simulink subsystem "MacPhersonFrntSolidAxleMidlRearSusp"  (R2023b)
settings: Solver=VariableStepAuto  StartTime=0.0  StopTime=10.0  RelTol=1e-3
undefined symbols (not defined in the file): PlntVehCGHgtAxl
libraries: sharedtransform x4, vehdynlibsuspension x2, autolibutils x2, matrix_library x1
settings Model: ModifiedByFormat=The MathWorks, Inc.  Creator=The MathWorks, Inc.  LastModifiedBy=The MathWorks, Inc.
settings OptimizationCC: ReuseModelBlockBuffer=off

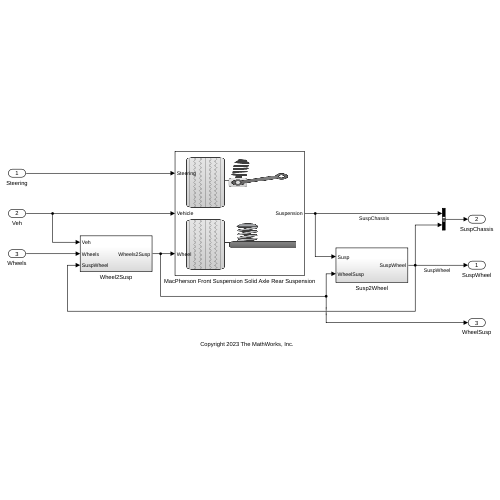
[thumbnail: Simulink's stored preview of the top-level diagram]
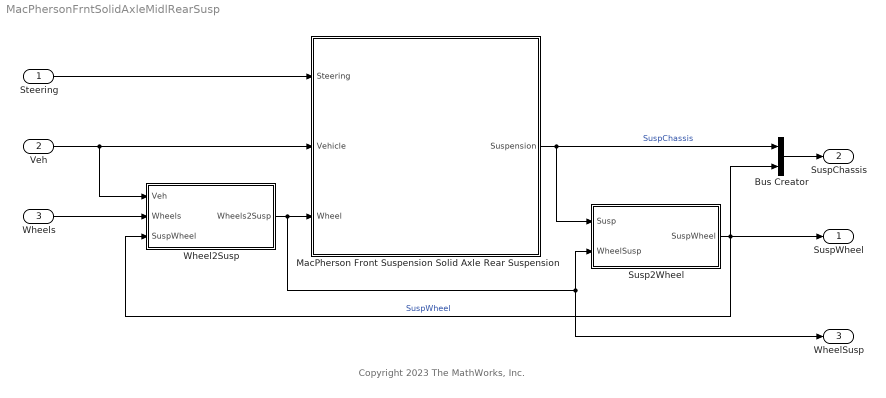
== system MacPhersonFrntSolidAxleMidlRearSusp ==
  note: Copyright 2023 The MathWorks, Inc.
  Steering : Inport
  Veh : Inport  Port=2
  Wheels : Inport  Port=3
  Bus Creator : BusCreator  Inputs=2
  MacPherson Front Suspension Solid Axle Rear Suspension : Subsystem  VariantControl=MacPherson Front Suspension Solid Axle Rear Suspension
      mask Display: image([imread('suspmacp.png');imread('suspsacoil.png')]);
  Susp2Wheel : Subsystem
  Wheel2Susp : Subsystem
  SuspWheel : Outport
  SuspChassis : Outport  Port=2
  WheelSusp : Outport  Port=3
  wires:
  Bus Creator/1 -> SuspChassis/1
  Wheel2Susp/1(Wheels2Susp) -> Susp2Wheel/2(WheelSusp), WheelSusp/1, MacPherson Front Suspension Solid Axle Rear Suspension/3(Wheel)
  Susp2Wheel/1(SuspWheel) -> SuspWheel/1, Bus Creator/2, Wheel2Susp/3(SuspWheel)  "SuspWheel"
  Wheels/1 -> Wheel2Susp/2(Wheels)
  Steering/1 -> MacPherson Front Suspension Solid Axle Rear Suspension/1(Steering)
  Veh/1 -> Wheel2Susp/1(Veh), MacPherson Front Suspension Solid Axle Rear Suspension/2(Vehicle)
  MacPherson Front Suspension Solid Axle Rear Suspension/1(Suspension) -> Susp2Wheel/1(Susp), Bus Creator/1  "SuspChassis"

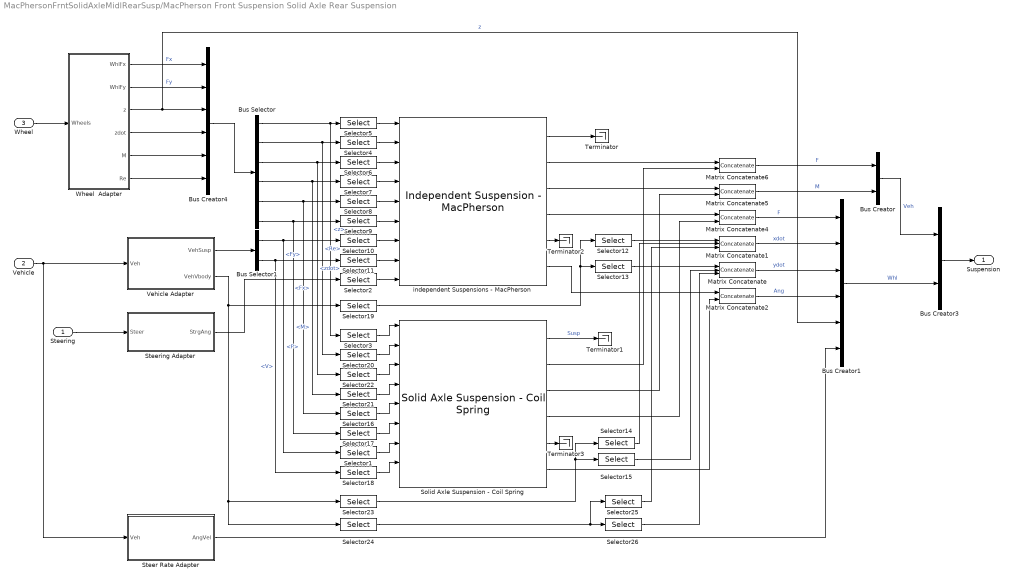
== system MacPhersonFrntSolidAxleMidlRearSusp/MacPherson Front Suspension Solid Axle Rear Suspension ==
  Steering : Inport
  Vehicle : Inport  Port=2
  Wheel : Inport  Port=3
  Bus Creator : BusCreator  Inputs=2
  Bus Creator1 : BusCreator  Inputs=6
  Bus Creator3 : BusCreator  Inputs=2
  Bus Creator4 : BusCreator  Inputs=6
  Bus Selector : BusSelector  OutputSignals=z,Re,zdot,Fx,Fy,M
  Bus Selector1 : BusSelector  OutputSignals=P,V
  Matrix Concatenate : Concatenate  NumInputs=3  Mode=Multidimensional array  ConcatenateDimension=2
  Matrix Concatenate1 : Concatenate  NumInputs=3  Mode=Multidimensional array  ConcatenateDimension=2
  Matrix Concatenate{2,4..6} (4 alike) : Concatenate  Mode=Multidimensional array  ConcatenateDimension=2
  Selector1 : Selector  NumberOfDimensions=2  IndexOptions=Select all,Index vector (dialog)  Indices=[1 2],[3 4 5 6]  OutputSizes=1,1
  Selector{9..11,19} (4 alike) : Selector  NumberOfDimensions=2  IndexOptions=Select all,Index vector (dialog)  Indices=[1 2],[1 2]  OutputSizes=1,1
  Selector12 : Selector  NumberOfDimensions=2  InputPortWidth=3  IndexOptions=Index vector (dialog),Select all  Indices=1,1  OutputSizes=1,1
  Selector13 : Selector  NumberOfDimensions=2  InputPortWidth=3  IndexOptions=Index vector (dialog),Select all  Indices=2,1  OutputSizes=1,1
  Selector14 : Selector  NumberOfDimensions=2  InputPortWidth=3  IndexOptions=Index vector (dialog),Select all  Indices=1,1  OutputSizes=1,1
  Selector15 : Selector  NumberOfDimensions=2  InputPortWidth=3  IndexOptions=Index vector (dialog),Select all  Indices=2,1  OutputSizes=1,1
  Selector{3,16,20..22} (5 alike) : Selector  IndexOptions=Index vector (dialog)  Indices=[3 4 5 6]  OutputSizes=1
  Selector17 : Selector  NumberOfDimensions=2  IndexOptions=Select all,Index vector (dialog)  Indices=[1 2],[3 4 5 6]  OutputSizes=1,1
  Selector18 : Selector  NumberOfDimensions=2  IndexOptions=Select all,Index vector (dialog)  Indices=[1 2],[3 4 5 6]  OutputSizes=1,1
  Selector2 : Selector  IndexOptions=Index vector (dialog)  Indices=[1 2]  OutputSizes=1
  Selector23 : Selector  NumberOfDimensions=2  IndexOptions=Select all,Index vector (dialog)  Indices=[1 2],[3 4]  OutputSizes=1,1
  Selector24 : Selector  NumberOfDimensions=2  IndexOptions=Select all,Index vector (dialog)  Indices=[1 2],[5 6]  OutputSizes=1,1
  Selector25 : Selector  NumberOfDimensions=2  InputPortWidth=3  IndexOptions=Index vector (dialog),Select all  Indices=1,1  OutputSizes=1,1
  Selector26 : Selector  NumberOfDimensions=2  InputPortWidth=3  IndexOptions=Index vector (dialog),Select all  Indices=2,1  OutputSizes=1,1
  Selector{4..8} (5 alike) : Selector  InputPortWidth=6  IndexOptions=Index vector (dialog)  Indices=[1 2]  OutputSizes=1
  Solid Axle Suspension - Coil Spring : vehdynlibsuspension/Solid Axle Suspension - Coil Spring  NumAxl=2  NumWhlsByAxl=[2 2]  StrgEnByAxl=[0 0]  WhlNumVec="[1  2  1  2]"  AxleNumVec="[1  1  2  2]"  SuspTypesByAxle="[1  1]"  SuspImage=suspsacoil.png  AxlIxx=PlntSpSARollInertia  AxlM=PlntSpSAAxleMass  TrackCoords="[zeros(1,4);1.575*[1 -1  1 -1]/2;zeros(1,4)]"  SuspCoords="[zeros(1,4);1.575*[1 -1  1 -1]/2;zeros(1,4)]"  KzWhlAxl=PlntSpSAAxleWheelStiffness  F0zWhlAxl=PlntSpSAAxleWheelPreload  CzWhlAxl=PlntSpSAAxleWheelDamping  IdealSuspEn=on  IdealSuspAxles="[1  2]"  Kz=PlntSpSAStiffness  F0z=PlntSpSAPreload  Cz=PlntSpSADamping  Hmax=PlntSpSAMaxHeight  Toe=PlntSpSAStatToe  RollStrgSlp=0.  ToeStrgSlp=0  Caster=PlntSpSAStatCaster  CasterHslp=0.  CasterStrgSlp=0.01  Camber=PlntSpSAStatCamber  CamberHslp=0.  CamberStrgSlp=0.01  StrgHgtSlp=0.1432  MappedSuspEn=off  MappedSuspAxles="[1  2]"  f_susp_axl_bp=[1 2]  f_susp_dz_bp=[-0.15 -0.14 -0.13 -0.12 -0.11 -0.10 -0.09 -0.08 -0.07 -0.06 -0.05 -0.04 -0.03 -0.02 -0.01 0.00 0.01 0.02 0.03 0.04 0.05 0.06 0.07 0.08 0.09 0.10 0.11 0.12 0.13 0.14 0.15]  f_susp_dzdot_bp=[-0.15 -0.14 -0.13 -0.12 -0.11 -0.10 -0.09 -0.08 -0.07 -0.06 -0.05 -0.04 -0.03 -0.02 -0.01 0.00 0.01 0.02 0.03 0.04 0.05 0.06 0.07 0.08 0.09 0.10 0.11 0.12 0.13 0.14 0.15]  f_susp_fmz=zeros(31,31,61,2,4)  f_susp_geom=zeros(31,61,2,3)  f_susp_strgdelta_bp=[-30,-29,-28,-27,-26,-25,-24,-23,-22,-21,-20,-19,-18,-17,-16,-15,-14,-13,-12,-11,-10,-9,-8,-7,-6,-5,-4,-3,-2,-1,0,1,2,3,4,5,6,7,8,9,10,11,12,13,14,15,16,17,18,19,20,21,22,23,24,25,26,27,28,29,30]
  Steer Rate Adapter : Subsystem
  Steering Adapter : Subsystem
  Terminator{,1..3} (4 alike) : Terminator
  Vehicle Adapter : Subsystem
  Wheel  Adapter : Subsystem
  independent Suspensions - MacPherson : vehdynlibsuspension/Independent Suspension - MacPherson  ActiveDampEn=off  NumAxl=1  NumWhlsByAxl=2  StrgEnByAxl=1  AntiSwayEnByAxl=1  WhlNumVec="[1  2]"  AxleNumVec="[1  1]"  SuspTypesByAxle=[1]  SuspImage=suspmacp.png  IdealSuspEn=on  IdealSuspAxles=[1]  Kz=PlntSpMSStiffness  F0z=PlntSpMSPreload  Cz=PlntSpMSDamping  Hmax=PlntSpMSMaxHeight  f_act_susp_cz=[10000 10000;10000 10000]  f_act_susp_duty_bpt=[0 1]  f_act_susp_zdot_bpt=[-1 1]  Toe=PlntSpMSStatToe  RollStrgSlp=0.  ToeStrgSlp=0.  Caster=PlntSpMSStatCaster  CasterHslp=0.  CasterStrgSlp=0.  Camber=PlntSpMSStatCamber  CamberHslp=0.  CamberStrgSlp=0.  StrgHgtSlp=PlntSpMSHeightVsSteer  MappedSuspEn=off  MappedSuspAxles="[1  2]"  f_susp_axl_bp=[1 2]  f_susp_dz_bp=[-0.15 -0.14 -0.13 -0.12 -0.11 -0.10 -0.09 -0.08 -0.07 -0.06 -0.05 -0.04 -0.03 -0.02 -0.01 0.00 0.01 0.02 0.03 0.04 0.05 0.06 0.07 0.08 0.09 0.10 0.11 0.12 0.13 0.14 0.15]  f_susp_dzdot_bp=[-0.15 -0.14 -0.13 -0.12 -0.11 -0.10 -0.09 -0.08 -0.07 -0.06 -0.05 -0.04 -0.03 -0.02 -0.01 0.00 0.01 0.02 0.03 0.04 0.05 0.06 0.07 0.08 0.09 0.10 0.11 0.12 0.13 0.14 0.15]  f_susp_fmz=zeros(31,31,61,2,4)  f_susp_geom=zeros(31,61,2,3)  f_susp_strgdelta_bp=[-30,-29,-28,-27,-26,-25,-24,-23,-22,-21,-20,-19,-18,-17,-16,-15,-14,-13,-12,-11,-10,-9,-8,-7,-6,-5,-4,-3,-2,-1,0,1,2,3,4,5,6,7,8,9,10,11,12,13,14,15,16,17,18,19,20,21,22,23,24,25,26,27,28,29,30]  AntiSwayR=PlntSpMSAntiSwayRadius  AntiSwayNtrlAng=PlntSpMSAntiSwayNeutralAngle  AntiSwayTrsK=PlntSpMSAntiSwayTorsionStiffness
  Suspension : Outport  VectorParamsAs1DForOutWhenUnconnected=off
  wires:
  Selector26/1 -> Matrix Concatenate/3
  Selector25/1 -> Matrix Concatenate1/3
  Selector24/1 -> Selector25/1, Selector26/1
  Selector23/1 -> Selector14/1, Selector15/1
  Selector19/1 -> Selector13/1, Selector12/1
  Solid Axle Suspension - Coil Spring/5 -> Terminator3/1
  independent Suspensions - MacPherson/5 -> Terminator2/1
  Steer Rate Adapter/1(AngVel) -> Bus Creator1/6
  Vehicle Adapter/2(VehVbody) -> Selector19/1, Selector23/1, Selector24/1
  Solid Axle Suspension - Coil Spring/1 -> Terminator1/1  "Susp"
  Bus Selector/3 -> Selector6/1, Selector22/1  "<zdot>"
  Selector22/1 -> Solid Axle Suspension - Coil Spring/3
  Vehicle/1 -> Steer Rate Adapter/1(Veh), Vehicle Adapter/1(Veh)
  Solid Axle Suspension - Coil Spring/3 -> Matrix Concatenate5/2
  Selector21/1 -> Solid Axle Suspension - Coil Spring/4
  Wheel  Adapter/6(Re) -> Bus Creator4/6
  Selector20/1 -> Solid Axle Suspension - Coil Spring/2
  Selector18/1 -> Solid Axle Suspension - Coil Spring/8
  Selector1/1 -> Solid Axle Suspension - Coil Spring/7
  Selector17/1 -> Solid Axle Suspension - Coil Spring/6
  Selector16/1 -> Solid Axle Suspension - Coil Spring/5
  Solid Axle Suspension - Coil Spring/2 -> Matrix Concatenate6/2
  Matrix Concatenate6/1 -> Bus Creator/1  "F"
  Matrix Concatenate5/1 -> Bus Creator/2  "M"
  Solid Axle Suspension - Coil Spring/4 -> Matrix Concatenate4/2
  Matrix Concatenate4/1 -> Bus Creator1/1  "F"
  Solid Axle Suspension - Coil Spring/6 -> Matrix Concatenate2/2
  Matrix Concatenate2/1 -> Bus Creator1/4  "Ang"
  Selector14/1 -> Matrix Concatenate1/2
  Matrix Concatenate1/1 -> Bus Creator1/2  "xdot"
  Selector15/1 -> Matrix Concatenate/2
  Selector13/1 -> Matrix Concatenate/1
  Selector11/1 -> independent Suspensions - MacPherson/8
  Selector10/1 -> independent Suspensions - MacPherson/7
  Selector9/1 -> independent Suspensions - MacPherson/6
  Selector8/1 -> independent Suspensions - MacPherson/5
  Selector7/1 -> independent Suspensions - MacPherson/4
  Selector6/1 -> independent Suspensions - MacPherson/3
  Selector5/1 -> independent Suspensions - MacPherson/1
  Selector4/1 -> independent Suspensions - MacPherson/2
  Selector3/1 -> Solid Axle Suspension - Coil Spring/1
  Selector2/1 -> independent Suspensions - MacPherson/9
  Bus Selector/2 -> Selector4/1, Selector20/1  "<Re>"
  Wheel  Adapter/5(M) -> Bus Creator4/5
  Wheel  Adapter/4(zdot) -> Bus Creator4/4
  Wheel  Adapter/3(z) -> Bus Creator4/3, Bus Creator1/5  "z"
  Wheel/1 -> Wheel  Adapter/1(Wheels)
  Wheel  Adapter/1(WhlFx) -> Bus Creator4/1  "Fx"
  Wheel  Adapter/2(WhlFy) -> Bus Creator4/2  "Fy"
  Bus Creator4/1 -> Bus Selector/1
  Steering Adapter/1(StrgAng) -> Selector2/1
  Bus Creator/1 -> Bus Creator3/1  "Veh"
  independent Suspensions - MacPherson/3 -> Matrix Concatenate5/1
  independent Suspensions - MacPherson/2 -> Matrix Concatenate6/1
  Vehicle Adapter/1(VehSusp) -> Bus Selector1/1
  Bus Selector/4 -> Selector21/1, Selector7/1  "<Fx>"
  independent Suspensions - MacPherson/1 -> Terminator/1
  independent Suspensions - MacPherson/4 -> Matrix Concatenate4/1
  Selector12/1 -> Matrix Concatenate1/1
  independent Suspensions - MacPherson/6 -> Matrix Concatenate2/1
  Matrix Concatenate/1 -> Bus Creator1/3  "ydot"
  Bus Selector1/1 -> Selector1/1, Selector10/1  "<P>"
  Steering/1 -> Steering Adapter/1(Steer)
  Bus Selector/1 -> Selector5/1, Selector3/1  "<z>"
  Bus Selector/5 -> Selector16/1, Selector8/1  "<Fy>"
  Bus Selector/6 -> Selector17/1, Selector9/1  "<M>"
  Bus Selector1/2 -> Selector18/1, Selector11/1  "<V>"
  Bus Creator1/1 -> Bus Creator3/2  "Whl"
  Bus Creator3/1 -> Suspension/1

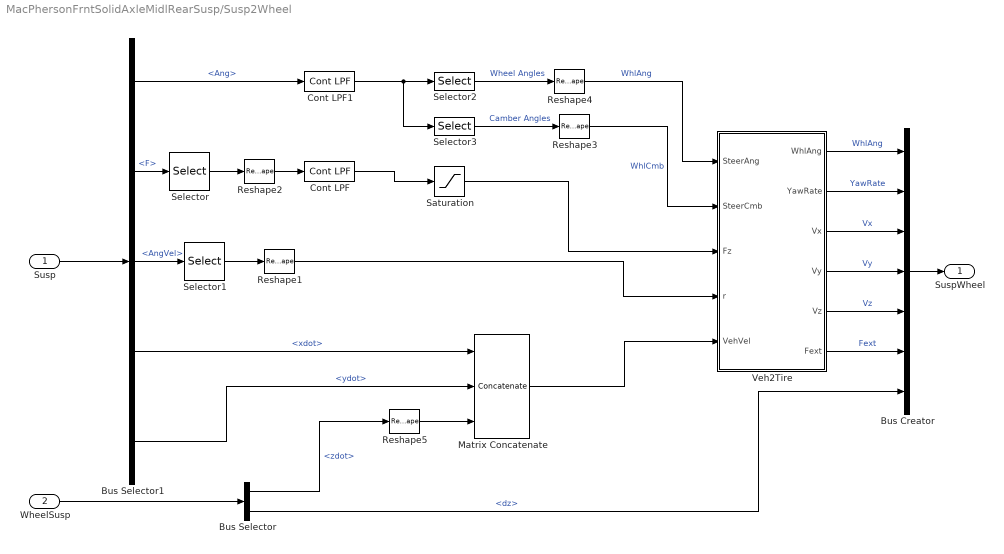
== system MacPhersonFrntSolidAxleMidlRearSusp/Susp2Wheel ==
  Susp : Inport
  WheelSusp : Inport  Port=2
  Bus Creator : BusCreator  Inputs=7
  Bus Selector : BusSelector  OutputSignals=SuspFrame.zdot,SuspFrame.dz
  Bus Selector1 : BusSelector  OutputSignals=Whl.Ang,Whl.F,Whl.AngVel,Whl.xdot,Whl.ydot
  Cont LPF : autolibutils/Cont LPF  wc=100*2*pi  AbsoluteTolerance=auto  aMode=2
  Cont LPF1 : autolibutils/Cont LPF  wc=100*2*pi  AbsoluteTolerance=auto  aMode=2
  Matrix Concatenate : Concatenate  NumInputs=3  Mode=Multidimensional array
  Reshape{1..4} (4 alike) : Reshape
  Reshape5 : Reshape  OutputDimensionality=Row vector (2-D)
  Saturation : Saturate  UpperLimit=inf  LowerLimit=-10*9.81*2000  ZeroCross=off
  Selector : Selector  NumberOfDimensions=2  InputPortWidth=3  IndexOptions=Index vector (dialog),Select all  Indices=[3],1  OutputSizes=1,1
  Selector1 : Selector  NumberOfDimensions=2  InputPortWidth=1  IndexOptions=Index vector (dialog),Select all  Indices=[3],1  OutputSizes=1,1
  Selector2 : Selector  NumberOfDimensions=2  InputPortWidth=3  IndexOptions=Index vector (dialog),Select all  Indices=3,1  OutputSizes=1,1
  Selector3 : Selector  NumberOfDimensions=2  InputPortWidth=3  IndexOptions=Index vector (dialog),Select all  Indices=1,1  OutputSizes=1,1
  Veh2Tire : Subsystem
  SuspWheel : Outport
  wires:
  Bus Creator/1 -> SuspWheel/1
  Bus Selector/1 -> Reshape5/1  "<zdot>"
  Veh2Tire/3(Vx) -> Bus Creator/3  "Vx"
  Veh2Tire/4(Vy) -> Bus Creator/4  "Vy"
  Susp/1 -> Bus Selector1/1
  Veh2Tire/5(Vz) -> Bus Creator/5  "Vz"
  Bus Selector1/1 -> Cont LPF1/1  "<Ang>"
  Reshape5/1 -> Matrix Concatenate/3
  WheelSusp/1 -> Bus Selector/1
  Cont LPF/1 -> Saturation/1
  Selector/1 -> Reshape2/1
  Matrix Concatenate/1 -> Veh2Tire/5(VehVel)
  Saturation/1 -> Veh2Tire/3(Fz)
  Selector1/1 -> Reshape1/1
  Veh2Tire/6(Fext) -> Bus Creator/6  "Fext"
  Bus Selector1/5 -> Matrix Concatenate/2  "<ydot>"
  Bus Selector1/3 -> Selector1/1  "<AngVel>"
  Bus Selector1/4 -> Matrix Concatenate/1  "<xdot>"
  Reshape4/1 -> Veh2Tire/1(SteerAng)  "WhlAng"
  Veh2Tire/1(WhlAng) -> Bus Creator/1  "WhlAng"
  Reshape3/1 -> Veh2Tire/2(SteerCmb)  "WhlCmb"
  Selector3/1 -> Reshape3/1  "Camber Angles"
  Reshape2/1 -> Cont LPF/1
  Selector2/1 -> Reshape4/1  "Wheel Angles"
  Reshape1/1 -> Veh2Tire/4(r)
  Cont LPF1/1 -> Selector3/1, Selector2/1
  Bus Selector1/2 -> Selector/1  "<F>"
  Veh2Tire/2(YawRate) -> Bus Creator/2  "YawRate"
  Bus Selector/2 -> Bus Creator/7  "<dz>"

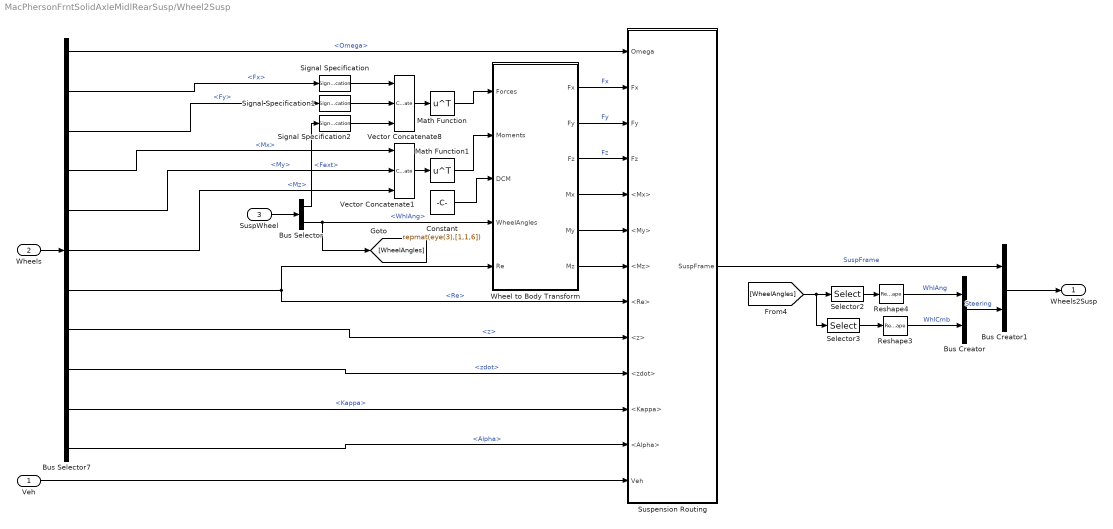
== system MacPhersonFrntSolidAxleMidlRearSusp/Wheel2Susp ==
  Veh : Inport
  Wheels : Inport  Port=2
  SuspWheel : Inport  Port=3
  Bus Creator : BusCreator  Inputs=2
  Bus Creator1 : BusCreator  Inputs=2
  Bus Selector : BusSelector  OutputSignals=Fext,WhlAng
  Bus Selector7 : BusSelector  OutputSignals=Wheels.Omega,Wheels.Fx,Wheels.Fy,Wheels.Mx,Wheels.My,Wheels.Mz,Wheels.Re,Wheels.z,Wheels.zdot,Wheels.Kappa,Wheels.Alpha
  Constant : Constant  Value=repmat(eye(3),[1,1,6])
  Math Function : Math  Operator=transpose  SignedPower=on
  Math Function1 : Math  Operator=transpose  SignedPower=on
  Reshape3 : Reshape
  Reshape4 : Reshape
  Selector2 : Selector  NumberOfDimensions=2  InputPortWidth=3  IndexOptions=Index vector (dialog),Select all  Indices=3,1  OutputSizes=1,1
  Selector3 : Selector  NumberOfDimensions=2  InputPortWidth=3  IndexOptions=Index vector (dialog),Select all  Indices=1,1  OutputSizes=1,1
  Signal Specification : SignalSpecification  Dimensions=6
  Signal Specification1 : SignalSpecification  Dimensions=6
  Signal Specification2 : SignalSpecification  Dimensions=6
  Suspension Routing : Subsystem
  Vector Concatenate1 : Concatenate  NumInputs=3  Mode=Multidimensional array  ConcatenateDimension=2
  Vector Concatenate8 : Concatenate  NumInputs=3  Mode=Multidimensional array  ConcatenateDimension=2
  Wheel to Body Transform : Subsystem
  Wheels2Susp : Outport  VectorParamsAs1DForOutWhenUnconnected=off
  wires:
  Bus Selector7/11 -> Suspension Routing/12(<Alpha>)  "<Alpha>"
  Bus Selector7/10 -> Suspension Routing/11(<Kappa>)  "<Kappa>"
  Bus Selector7/9 -> Suspension Routing/10(<zdot>)  "<zdot>"
  Bus Selector7/8 -> Suspension Routing/9(<z>)  "<z>"
  Bus Selector7/7 -> Suspension Routing/8(<Re>), Wheel to Body Transform/5(Re)  "<Re>"
  Bus Selector7/6 -> Vector Concatenate1/3  "<Mz>"
  Bus Selector7/5 -> Vector Concatenate1/2  "<My>"
  Bus Selector7/4 -> Vector Concatenate1/1  "<Mx>"
  Bus Selector7/3 -> Signal Specification1/1  "<Fy>"
  Bus Selector7/2 -> Signal Specification/1  "<Fx>"
  Bus Selector7/1 -> Suspension Routing/1(Omega)  "<Omega>"
  Constant/1 -> Wheel to Body Transform/3(DCM)
  Math Function1/1 -> Wheel to Body Transform/2(Moments)
  Vector Concatenate1/1 -> Math Function1/1
  Wheel to Body Transform/6(Mz) -> Suspension Routing/7(<Mz>)
  Wheel to Body Transform/5(My) -> Suspension Routing/6(<My>)
  Wheel to Body Transform/4(Mx) -> Suspension Routing/5(<Mx>)
  Selector3/1 -> Reshape3/1
  [WheelAngles] -> Selector3/1, Selector2/1
  Selector2/1 -> Reshape4/1
  Signal Specification2/1 -> Vector Concatenate8/3
  Bus Selector/1 -> Signal Specification2/1  "<Fext>"
  SuspWheel/1 -> Bus Selector/1
  Wheel to Body Transform/2(Fy) -> Suspension Routing/3(Fy)  "Fy"
  Wheel to Body Transform/1(Fx) -> Suspension Routing/2(Fx)  "Fx"
  Vector Concatenate8/1 -> Math Function/1
  Math Function/1 -> Wheel to Body Transform/1(Forces)
  Wheels/1 -> Bus Selector7/1
  Bus Selector/2 -> Wheel to Body Transform/4(WheelAngles), [WheelAngles]  "<WhlAng>"
  Wheel to Body Transform/3(Fz) -> Suspension Routing/4(Fz)  "Fz"
  Reshape4/1 -> Bus Creator/1  "WhlAng"
  Bus Creator1/1 -> Wheels2Susp/1
  Suspension Routing/1(SuspFrame) -> Bus Creator1/1  "SuspFrame"
  Reshape3/1 -> Bus Creator/2  "WhlCmb"
  Bus Creator/1 -> Bus Creator1/2  "Steering"
  Veh/1 -> Suspension Routing/13(Veh)
  Signal Specification/1 -> Vector Concatenate8/1
  Signal Specification1/1 -> Vector Concatenate8/2

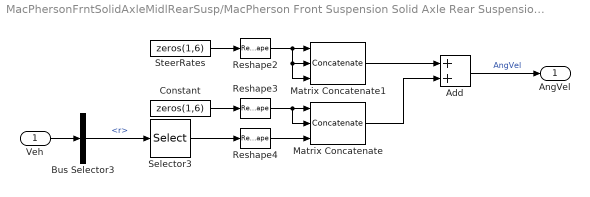
== system MacPhersonFrntSolidAxleMidlRearSusp/MacPherson Front Suspension Solid Axle Rear Suspension/Steer Rate Adapter ==
  Veh : Inport
  Add : Sum
  Bus Selector3 : BusSelector  OutputSignals=BdyFrm.Cg.AngVel.r
  Constant : Constant  Value=zeros(1,6)  SampleTime=-1
  Matrix Concatenate : Concatenate  NumInputs=3  Mode=Multidimensional array
  Matrix Concatenate1 : Concatenate  NumInputs=3  Mode=Multidimensional array
  Reshape2 : Reshape  OutputDimensionality=Row vector (2-D)
  Reshape3 : Reshape  OutputDimensionality=Row vector (2-D)
  Reshape4 : Reshape  OutputDimensionality=Row vector (2-D)
  Selector3 : Selector  InputPortWidth=1  IndexOptions=Index vector (dialog)  Indices=[1 1 1 1 1 1]  OutputSizes=1
  SteerRates : Constant  Value=zeros(1,6)  SampleTime=-1
  AngVel : Outport  VectorParamsAs1DForOutWhenUnconnected=off
  wires:
  Add/1 -> AngVel/1  "AngVel"
  Veh/1 -> Bus Selector3/1
  Matrix Concatenate1/1 -> Add/1
  Reshape3/1 -> Matrix Concatenate/1, Matrix Concatenate/2
  Reshape4/1 -> Matrix Concatenate/3
  SteerRates/1 -> Reshape2/1
  Matrix Concatenate/1 -> Add/2
  Bus Selector3/1 -> Selector3/1  "<r>"
  Selector3/1 -> Reshape4/1
  Constant/1 -> Reshape3/1
  Reshape2/1 -> Matrix Concatenate1/2, Matrix Concatenate1/3, Matrix Concatenate1/1

== system MacPhersonFrntSolidAxleMidlRearSusp/MacPherson Front Suspension Solid Axle Rear Suspension/Steering Adapter ==
  Steer : Inport
  Reshape1 : Reshape  OutputDimensionality=Row vector (2-D)
  Selector : Selector  IndexOptions=Index vector (dialog)  Indices=[1 2]  OutputSizes=1
  StrgAng : Outport  VectorParamsAs1DForOutWhenUnconnected=off
  wires:
  Selector/1 -> Reshape1/1
  Steer/1 -> Selector/1
  Reshape1/1 -> StrgAng/1

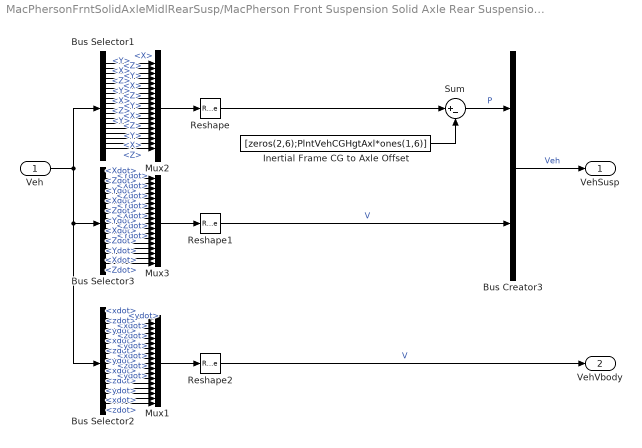
== system MacPhersonFrntSolidAxleMidlRearSusp/MacPherson Front Suspension Solid Axle Rear Suspension/Vehicle Adapter ==
  Veh : Inport
  Bus Creator3 : BusCreator  Inputs=2
  Bus Selector1 : BusSelector  OutputSignals=InertFrm.FrntAxl.Lft.Disp.X,InertFrm.FrntAxl.Lft.Disp.Y,InertFrm.FrntAxl.Lft.Disp.Z,InertFrm.FrntAxl.Rght.Disp.X,InertFrm.FrntAxl.Rght.Disp.Y,InertFrm.FrntAxl.Rght.Disp.Z,InertFrm.MidlAxl.Lft.Disp.X,InertFrm.MidlAxl.Lft.Disp.Y,InertFrm.MidlAxl.Lft.Disp.Z,InertFrm.MidlAxl.Rght.Disp.X,InertFrm.MidlAxl.Rght.Disp.Y,InertFrm.MidlAxl.Rght.Disp.Z,InertFrm.RearAxl.Lft.Disp.X,InertFrm.RearAxl.Lft.Disp.Y,InertFrm.RearAxl.Lft.Disp.Z,InertFrm.RearAxl.Rght.Disp.X,InertFrm.RearAxl.Rght.Disp.Y,InertFrm.RearAxl.Rght.Disp.Z
  Bus Selector2 : BusSelector  OutputSignals=BdyFrm.FrntAxl.Lft.Vel.xdot,BdyFrm.FrntAxl.Lft.Vel.ydot,BdyFrm.FrntAxl.Lft.Vel.zdot,BdyFrm.FrntAxl.Rght.Vel.xdot,BdyFrm.FrntAxl.Rght.Vel.ydot,BdyFrm.FrntAxl.Rght.Vel.zdot,BdyFrm.MidlAxl.Lft.Vel.xdot,BdyFrm.MidlAxl.Lft.Vel.ydot,BdyFrm.MidlAxl.Lft.Vel.zdot,BdyFrm.MidlAxl.Rght.Vel.xdot,BdyFrm.MidlAxl.Rght.Vel.ydot,BdyFrm.MidlAxl.Rght.Vel.zdot,BdyFrm.RearAxl.Lft.Vel.xdot,BdyFrm.RearAxl.Lft.Vel.ydot,BdyFrm.RearAxl.Lft.Vel.zdot,BdyFrm.RearAxl.Rght.Vel.xdot,BdyFrm.RearAxl.Rght.Vel.ydot,BdyFrm.RearAxl.Rght.Vel.zdot
  Bus Selector3 : BusSelector  OutputSignals=InertFrm.FrntAxl.Lft.Vel.Xdot,InertFrm.FrntAxl.Lft.Vel.Ydot,InertFrm.FrntAxl.Lft.Vel.Zdot,InertFrm.FrntAxl.Rght.Vel.Xdot,InertFrm.FrntAxl.Rght.Vel.Ydot,InertFrm.FrntAxl.Rght.Vel.Zdot,InertFrm.MidlAxl.Lft.Vel.Xdot,InertFrm.MidlAxl.Lft.Vel.Ydot,InertFrm.MidlAxl.Lft.Vel.Zdot,InertFrm.MidlAxl.Rght.Vel.Xdot,InertFrm.MidlAxl.Rght.Vel.Ydot,InertFrm.MidlAxl.Rght.Vel.Zdot,InertFrm.RearAxl.Lft.Vel.Xdot,InertFrm.RearAxl.Lft.Vel.Ydot,InertFrm.RearAxl.Lft.Vel.Zdot,InertFrm.RearAxl.Rght.Vel.Xdot,InertFrm.RearAxl.Rght.Vel.Ydot,InertFrm.RearAxl.Rght.Vel.Zdot
  Inertial Frame CG to Axle Offset : Constant  Value=[zeros(2,6);PlntVehCGHgtAxl*ones(1,6)]  SampleTime=-1
  Mux1 : Mux  Inputs=18
  Mux2 : Mux  Inputs=18
  Mux3 : Mux  Inputs=18
  Reshape : Reshape  OutputDimensionality=Customize  OutputDimensions=[3,6]
  Reshape1 : Reshape  OutputDimensionality=Customize  OutputDimensions=[3,6]
  Reshape2 : Reshape  OutputDimensionality=Customize  OutputDimensions=[3,6]
  Sum : Sum  Inputs=|+-
  VehSusp : Outport  VectorParamsAs1DForOutWhenUnconnected=off
  VehVbody : Outport  Port=2  VectorParamsAs1DForOutWhenUnconnected=off
  wires:
  Bus Selector2/18 -> Mux1/18  "<zdot>"
  Bus Selector2/17 -> Mux1/17  "<ydot>"
  Bus Selector2/16 -> Mux1/16  "<xdot>"
  Bus Selector2/15 -> Mux1/15  "<zdot>"
  Bus Selector2/14 -> Mux1/14  "<ydot>"
  Bus Selector2/13 -> Mux1/13  "<xdot>"
  Bus Selector2/12 -> Mux1/12  "<zdot>"
  Bus Selector2/11 -> Mux1/11  "<ydot>"
  Bus Selector2/10 -> Mux1/10  "<xdot>"
  Bus Selector2/9 -> Mux1/9  "<zdot>"
  Bus Selector2/8 -> Mux1/8  "<ydot>"
  Bus Selector2/7 -> Mux1/7  "<xdot>"
  Bus Selector2/6 -> Mux1/6  "<zdot>"
  Bus Selector2/5 -> Mux1/5  "<ydot>"
  Bus Selector2/4 -> Mux1/4  "<xdot>"
  Bus Selector2/3 -> Mux1/3  "<zdot>"
  Bus Selector2/2 -> Mux1/2  "<ydot>"
  Bus Selector2/1 -> Mux1/1  "<xdot>"
  Bus Selector3/18 -> Mux3/18  "<Zdot>"
  Bus Selector3/17 -> Mux3/17  "<Ydot>"
  Bus Selector3/16 -> Mux3/16  "<Xdot>"
  Bus Selector3/15 -> Mux3/15  "<Zdot>"
  Bus Selector3/14 -> Mux3/14  "<Ydot>"
  Bus Selector3/13 -> Mux3/13  "<Xdot>"
  Bus Selector3/12 -> Mux3/12  "<Zdot>"
  Bus Selector3/11 -> Mux3/11  "<Ydot>"
  Bus Selector3/10 -> Mux3/10  "<Xdot>"
  Bus Selector3/9 -> Mux3/9  "<Zdot>"
  Bus Selector3/8 -> Mux3/8  "<Ydot>"
  Bus Selector3/7 -> Mux3/7  "<Xdot>"
  Bus Selector3/6 -> Mux3/6  "<Zdot>"
  Bus Selector3/5 -> Mux3/5  "<Ydot>"
  Bus Selector3/4 -> Mux3/4  "<Xdot>"
  Bus Selector3/3 -> Mux3/3  "<Zdot>"
  Bus Selector3/2 -> Mux3/2  "<Ydot>"
  Bus Selector3/1 -> Mux3/1  "<Xdot>"
  Bus Selector1/18 -> Mux2/18  "<Z>"
  Bus Selector1/17 -> Mux2/17  "<Y>"
  Bus Selector1/16 -> Mux2/16  "<X>"
  Bus Selector1/15 -> Mux2/15  "<Z>"
  Bus Selector1/14 -> Mux2/14  "<Y>"
  Bus Selector1/13 -> Mux2/13  "<X>"
  Bus Selector1/12 -> Mux2/12  "<Z>"
  Bus Selector1/11 -> Mux2/11  "<Y>"
  Bus Selector1/10 -> Mux2/10  "<X>"
  Bus Selector1/9 -> Mux2/9  "<Z>"
  Bus Selector1/8 -> Mux2/8  "<Y>"
  Bus Selector1/7 -> Mux2/7  "<X>"
  Bus Selector1/6 -> Mux2/6  "<Z>"
  Bus Selector1/5 -> Mux2/5  "<Y>"
  Bus Selector1/4 -> Mux2/4  "<X>"
  Bus Selector1/3 -> Mux2/3  "<Z>"
  Bus Selector1/2 -> Mux2/2  "<Y>"
  Bus Selector1/1 -> Mux2/1  "<X>"
  Reshape1/1 -> Bus Creator3/2  "V"
  Mux3/1 -> Reshape1/1
  Sum/1 -> Bus Creator3/1  "P"
  Inertial Frame CG to Axle Offset/1 -> Sum/2
  Mux2/1 -> Reshape/1
  Mux1/1 -> Reshape2/1
  Reshape/1 -> Sum/1
  Bus Creator3/1 -> VehSusp/1  "Veh"
  Reshape2/1 -> VehVbody/1  "V"
  Veh/1 -> Bus Selector1/1, Bus Selector2/1, Bus Selector3/1

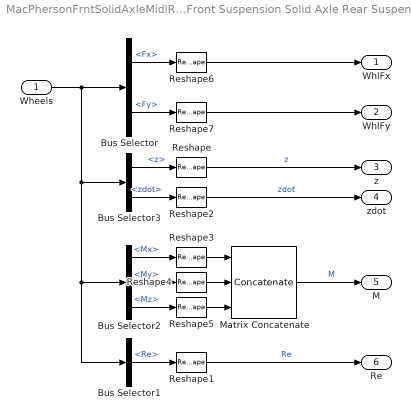
== system MacPhersonFrntSolidAxleMidlRearSusp/MacPherson Front Suspension Solid Axle Rear Suspension/Wheel  Adapter ==
  Wheels : Inport
  Bus Selector : BusSelector  OutputSignals=SuspFrame.Fx,SuspFrame.Fy
  Bus Selector1 : BusSelector  OutputSignals=SuspFrame.Re
  Bus Selector2 : BusSelector  OutputSignals=SuspFrame.Mx,SuspFrame.My,SuspFrame.Mz
  Bus Selector3 : BusSelector  OutputSignals=SuspFrame.z,SuspFrame.zdot
  Matrix Concatenate : Concatenate  NumInputs=3  Mode=Multidimensional array
  Reshape{,1..7} (8 alike) : Reshape  OutputDimensionality=Row vector (2-D)
  WhlFx : Outport  VectorParamsAs1DForOutWhenUnconnected=off
  WhlFy : Outport  Port=2  VectorParamsAs1DForOutWhenUnconnected=off
  z : Outport  Port=3  VectorParamsAs1DForOutWhenUnconnected=off
  zdot : Outport  Port=4  VectorParamsAs1DForOutWhenUnconnected=off
  M : Outport  Port=5  VectorParamsAs1DForOutWhenUnconnected=off
  Re : Outport  Port=6  VectorParamsAs1DForOutWhenUnconnected=off
  wires:
  Reshape/1 -> z/1  "z"
  Matrix Concatenate/1 -> M/1  "M"
  Reshape5/1 -> Matrix Concatenate/3
  Reshape4/1 -> Matrix Concatenate/2
  Reshape3/1 -> Matrix Concatenate/1
  Bus Selector2/3 -> Reshape5/1  "<Mz>"
  Bus Selector2/2 -> Reshape4/1  "<My>"
  Bus Selector2/1 -> Reshape3/1  "<Mx>"
  Reshape1/1 -> Re/1  "Re"
  Bus Selector1/1 -> Reshape1/1  "<Re>"
  Reshape2/1 -> zdot/1  "zdot"
  Bus Selector3/2 -> Reshape2/1  "<zdot>"
  Wheels/1 -> Bus Selector/1, Bus Selector3/1, Bus Selector2/1, Bus Selector1/1
  Bus Selector3/1 -> Reshape/1  "<z>"
  Bus Selector/2 -> Reshape7/1  "<Fy>"
  Bus Selector/1 -> Reshape6/1  "<Fx>"
  Reshape6/1 -> WhlFx/1
  Reshape7/1 -> WhlFy/1

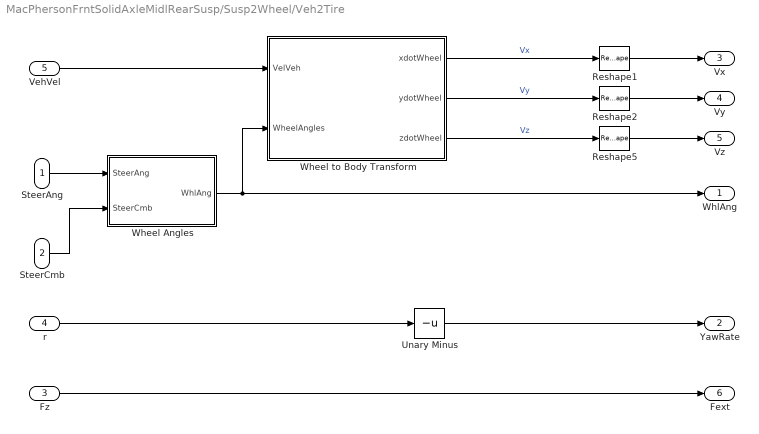
== system MacPhersonFrntSolidAxleMidlRearSusp/Susp2Wheel/Veh2Tire ==
  SteerAng : Inport
  SteerCmb : Inport  Port=2
  Fz : Inport  Port=3
  r : Inport  Port=4
  VehVel : Inport  Port=5
  Reshape1 : Reshape
  Reshape2 : Reshape
  Reshape5 : Reshape
  Unary Minus : UnaryMinus
  Wheel Angles : Subsystem
  Wheel to Body Transform : Subsystem
  WhlAng : Outport  Unit=rad  VectorParamsAs1DForOutWhenUnconnected=off
  YawRate : Outport  Port=2  Unit=rad/s  VectorParamsAs1DForOutWhenUnconnected=off
  Vx : Outport  Port=3  Unit=m/s  VectorParamsAs1DForOutWhenUnconnected=off
  Vy : Outport  Port=4  Unit=m/s  VectorParamsAs1DForOutWhenUnconnected=off
  Vz : Outport  Port=5  Unit=m/s  VectorParamsAs1DForOutWhenUnconnected=off
  Fext : Outport  Port=6  Unit=N  VectorParamsAs1DForOutWhenUnconnected=off
  wires:
  Fz/1 -> Fext/1
  Wheel to Body Transform/1(xdotWheel) -> Reshape1/1  "Vx"
  Wheel to Body Transform/2(ydotWheel) -> Reshape2/1  "Vy"
  SteerAng/1 -> Wheel Angles/1(SteerAng)
  r/1 -> Unary Minus/1
  VehVel/1 -> Wheel to Body Transform/1(VelVeh)
  Wheel to Body Transform/3(zdotWheel) -> Reshape5/1  "Vz"
  Unary Minus/1 -> YawRate/1
  Wheel Angles/1("WhlAng ") -> WhlAng/1, Wheel to Body Transform/2(WheelAngles)
  Reshape1/1 -> Vx/1
  Reshape2/1 -> Vy/1
  Reshape5/1 -> Vz/1
  SteerCmb/1 -> Wheel Angles/2(SteerCmb)

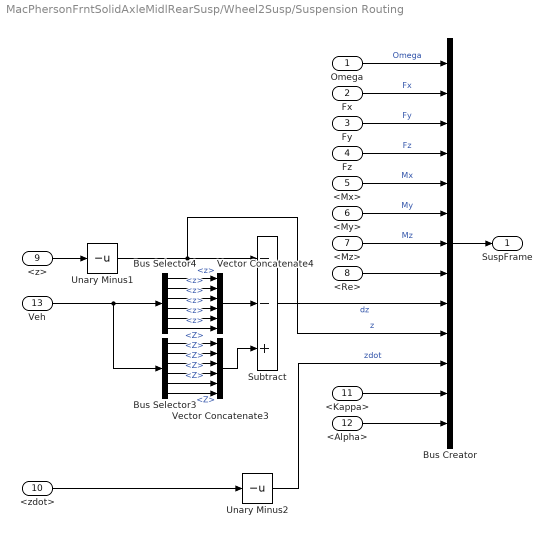
== system MacPhersonFrntSolidAxleMidlRearSusp/Wheel2Susp/Suspension Routing ==
  Omega : Inport
  Fx : Inport  Port=2
  Fy : Inport  Port=3
  Fz : Inport  Port=4
  <Mx> : Inport  Port=5
  <My> : Inport  Port=6
  <Mz> : Inport  Port=7
  <Re> : Inport  Port=8
  <z> : Inport  Port=9
  <zdot> : Inport  Port=10
  <Kappa> : Inport  Port=11
  <Alpha> : Inport  Port=12
  Veh : Inport  Port=13
  Bus Creator : BusCreator  Inputs=13
  Bus Selector3 : BusSelector  OutputSignals=InertFrm.FrntAxl.Lft.Disp.Z,InertFrm.FrntAxl.Rght.Disp.Z,InertFrm.MidlAxl.Lft.Disp.Z,InertFrm.MidlAxl.Rght.Disp.Z,InertFrm.RearAxl.Lft.Disp.Z,InertFrm.RearAxl.Rght.Disp.Z
  Bus Selector4 : BusSelector  OutputSignals=BdyFrm.FrntAxl.Lft.Disp.z,BdyFrm.FrntAxl.Rght.Disp.z,BdyFrm.MidlAxl.Lft.Disp.z,BdyFrm.MidlAxl.Rght.Disp.z,BdyFrm.RearAxl.Lft.Disp.z,BdyFrm.RearAxl.Rght.Disp.z
  Subtract : Sum  Inputs=--+
  Unary Minus1 : UnaryMinus
  Unary Minus2 : UnaryMinus
  Vector Concatenate3 : Concatenate  NumInputs=6
  Vector Concatenate4 : Concatenate  NumInputs=6
  SuspFrame : Outport  VectorParamsAs1DForOutWhenUnconnected=off
  wires:
  Bus Selector3/4 -> Vector Concatenate3/4  "<Z>"
  Bus Selector3/3 -> Vector Concatenate3/3  "<Z>"
  Bus Selector4/4 -> Vector Concatenate4/4  "<z>"
  Bus Selector4/3 -> Vector Concatenate4/3  "<z>"
  <Re>/1 -> Bus Creator/8
  Unary Minus1/1 -> Subtract/1, Bus Creator/10  "z"
  Fz/1 -> Bus Creator/4  "Fz"
  <zdot>/1 -> Unary Minus2/1
  <Mz>/1 -> Bus Creator/7  "Mz"
  Unary Minus2/1 -> Bus Creator/11  "zdot"
  <z>/1 -> Unary Minus1/1
  Bus Creator/1 -> SuspFrame/1
  Fy/1 -> Bus Creator/3  "Fy"
  Omega/1 -> Bus Creator/1  "Omega"
  Fx/1 -> Bus Creator/2  "Fx"
  <Kappa>/1 -> Bus Creator/12
  <Mx>/1 -> Bus Creator/5  "Mx"
  <My>/1 -> Bus Creator/6  "My"
  <Alpha>/1 -> Bus Creator/13
  Veh/1 -> Bus Selector3/1, Bus Selector4/1
  Bus Selector3/6 -> Vector Concatenate3/6  "<Z>"
  Subtract/1 -> Bus Creator/9  "dz"
  Bus Selector4/1 -> Vector Concatenate4/1  "<z>"
  Bus Selector3/1 -> Vector Concatenate3/1  "<Z>"
  Vector Concatenate3/1 -> Subtract/3
  Vector Concatenate4/1 -> Subtract/2
  Bus Selector4/2 -> Vector Concatenate4/2  "<z>"
  Bus Selector3/5 -> Vector Concatenate3/5  "<Z>"
  Bus Selector3/2 -> Vector Concatenate3/2  "<Z>"
  Bus Selector4/6 -> Vector Concatenate4/6  "<z>"
  Bus Selector4/5 -> Vector Concatenate4/5  "<z>"

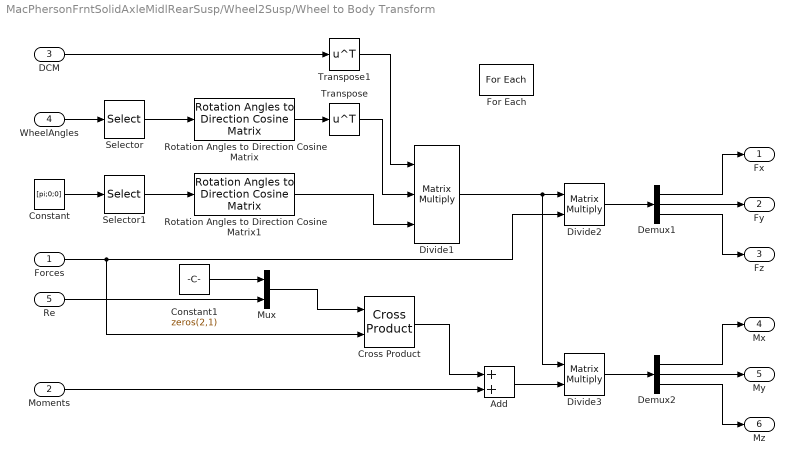
== system MacPhersonFrntSolidAxleMidlRearSusp/Wheel2Susp/Wheel to Body Transform ==
  Forces : Inport  PortDimensions=[3,1]  Partition=on  PartitionDimension=2  PartitionWidth=1  PartitionOffset=0
  Moments : Inport  Port=2  PortDimensions=[3,1]  Partition=on  PartitionDimension=2  PartitionWidth=1  PartitionOffset=0
  DCM : Inport  Port=3  Partition=on  PartitionDimension=3  PartitionWidth=1  PartitionOffset=0
  WheelAngles : Inport  Port=4  Partition=on  PartitionDimension=2  PartitionWidth=1  PartitionOffset=0
  Re : Inport  Port=5  Partition=on  PartitionDimension=1  PartitionWidth=1  PartitionOffset=0
  Add : Sum
  Constant : Constant  Value=[pi;0;0]
  Constant1 : Constant  Value=zeros(2,1)
  Cross Product : matrix_library/Cross Product
  Demux1 : Demux  Outputs=3
  Demux2 : Demux  Outputs=3
  Divide1 : Product  Inputs=***  Multiplication=Matrix(*)
  Divide2 : Product  Inputs=**  Multiplication=Matrix(*)
  Divide3 : Product  Inputs=**  Multiplication=Matrix(*)
  For Each : ForEach  DisableCoverage=on
  Mux : Mux  Inputs=2
  Rotation Angles to Direction Cosine Matrix : sharedtransform/Rotation Angles to Direction Cosine Matrix  rotationOrder=ZYX  aMode=2
  Rotation Angles to Direction Cosine Matrix1 : sharedtransform/Rotation Angles to Direction Cosine Matrix  rotationOrder=ZYX  aMode=2
  Selector : Selector  InputPortWidth=3  IndexOptions=Index vector (dialog)  Indices=[3 2 1]  OutputSizes=1
  Selector1 : Selector  InputPortWidth=3  IndexOptions=Index vector (dialog)  Indices=[3 2 1]  OutputSizes=1
  Transpose : Math  Operator=transpose
  Transpose1 : Math  Operator=transpose
  Fx : Outport  ConcatenationDimension=1  VectorParamsAs1DForOutWhenUnconnected=off
  Fy : Outport  Port=2  ConcatenationDimension=1  VectorParamsAs1DForOutWhenUnconnected=off
  Fz : Outport  Port=3  ConcatenationDimension=1  VectorParamsAs1DForOutWhenUnconnected=off
  Mx : Outport  Port=4  ConcatenationDimension=1  VectorParamsAs1DForOutWhenUnconnected=off
  My : Outport  Port=5  ConcatenationDimension=1  VectorParamsAs1DForOutWhenUnconnected=off
  Mz : Outport  Port=6  ConcatenationDimension=1  VectorParamsAs1DForOutWhenUnconnected=off
  wires:
  Constant1/1 -> Mux/1
  Re/1 -> Mux/2
  Mux/1 -> Cross Product/1
  Cross Product/1 -> Add/1
  Add/1 -> Divide3/2
  Demux2/1 -> Mx/1
  Demux2/2 -> My/1
  Demux2/3 -> Mz/1
  Moments/1 -> Add/2
  Divide1/1 -> Divide2/1, Divide3/1
  Divide3/1 -> Demux2/1
  Divide2/1 -> Demux1/1
  Transpose1/1 -> Divide1/1
  DCM/1 -> Transpose1/1
  Transpose/1 -> Divide1/2
  Constant/1 -> Selector1/1
  Selector1/1 -> Rotation Angles to Direction Cosine Matrix1/1
  Rotation Angles to Direction Cosine Matrix1/1 -> Divide1/3
  Selector/1 -> Rotation Angles to Direction Cosine Matrix/1
  WheelAngles/1 -> Selector/1
  Forces/1 -> Cross Product/2, Divide2/2
  Rotation Angles to Direction Cosine Matrix/1 -> Transpose/1
  Demux1/3 -> Fz/1
  Demux1/2 -> Fy/1
  Demux1/1 -> Fx/1

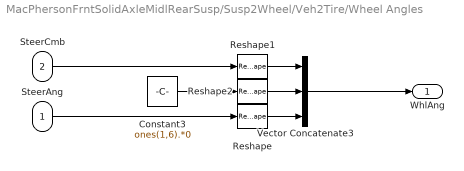
== system MacPhersonFrntSolidAxleMidlRearSusp/Susp2Wheel/Veh2Tire/Wheel Angles ==
  SteerAng : Inport
  SteerCmb : Inport  Port=2
  Constant3 : Constant  Value=ones(1,6).*0  SampleTime=-1
  Reshape : Reshape  OutputDimensionality=Row vector (2-D)
  Reshape1 : Reshape  OutputDimensionality=Row vector (2-D)
  Reshape2 : Reshape  OutputDimensionality=Row vector (2-D)
  Vector Concatenate3 : Concatenate  NumInputs=3  Mode=Multidimensional array
  "WhlAng " : Outport  VectorParamsAs1DForOutWhenUnconnected=off
  wires:
  Constant3/1 -> Reshape2/1
  Vector Concatenate3/1 -> "WhlAng "/1
  Reshape/1 -> Vector Concatenate3/3
  Reshape1/1 -> Vector Concatenate3/1
  SteerCmb/1 -> Reshape1/1
  Reshape2/1 -> Vector Concatenate3/2
  SteerAng/1 -> Reshape/1

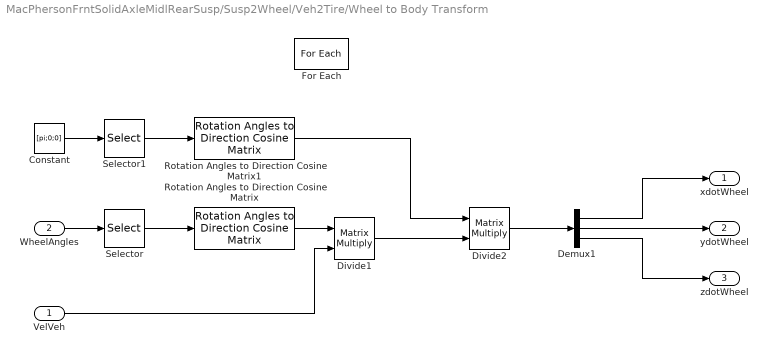
== system MacPhersonFrntSolidAxleMidlRearSusp/Susp2Wheel/Veh2Tire/Wheel to Body Transform ==
  VelVeh : Inport  Partition=on  PartitionDimension=2  PartitionWidth=1  PartitionOffset=0
  WheelAngles : Inport  Port=2  Partition=on  PartitionDimension=2  PartitionWidth=1  PartitionOffset=0
  Constant : Constant  Value=[pi;0;0]  SampleTime=-1
  Demux1 : Demux  Outputs=3
  Divide1 : Product  Inputs=**  Multiplication=Matrix(*)
  Divide2 : Product  Inputs=**  Multiplication=Matrix(*)
  For Each : ForEach  DisableCoverage=on
  Rotation Angles to Direction Cosine Matrix : sharedtransform/Rotation Angles to Direction Cosine Matrix  rotationOrder=ZYX  aMode=2
  Rotation Angles to Direction Cosine Matrix1 : sharedtransform/Rotation Angles to Direction Cosine Matrix  rotationOrder=ZYX  aMode=2
  Selector : Selector  InputPortWidth=3  IndexOptions=Index vector (dialog)  Indices=[3 2 1]  OutputSizes=1
  Selector1 : Selector  InputPortWidth=3  IndexOptions=Index vector (dialog)  Indices=[3 2 1]  OutputSizes=1
  xdotWheel : Outport  ConcatenationDimension=1  VectorParamsAs1DForOutWhenUnconnected=off
  ydotWheel : Outport  Port=2  ConcatenationDimension=1  VectorParamsAs1DForOutWhenUnconnected=off
  zdotWheel : Outport  Port=3  ConcatenationDimension=1  VectorParamsAs1DForOutWhenUnconnected=off
  wires:
  Divide2/1 -> Demux1/1
  Demux1/1 -> xdotWheel/1
  Demux1/2 -> ydotWheel/1
  Demux1/3 -> zdotWheel/1
  Rotation Angles to Direction Cosine Matrix/1 -> Divide1/1
  VelVeh/1 -> Divide1/2
  WheelAngles/1 -> Selector/1
  Selector/1 -> Rotation Angles to Direction Cosine Matrix/1
  Selector1/1 -> Rotation Angles to Direction Cosine Matrix1/1
  Rotation Angles to Direction Cosine Matrix1/1 -> Divide2/1
  Divide1/1 -> Divide2/2
  Constant/1 -> Selector1/1
